simulink model "xTyTbeta1beta2"  (Simulink 10.0)
settings: Solver=FixedStepDiscrete  StartTime=0.0  StopTime=TF  FixedStep=5e-2  RelTol=1e-4  EnableMultiTasking=on
values from neighbouring files (symbols this model uses):
  Lb1 = 0.3    [s_robot_planare.m]
  Lb2 = 0.4    [s_robot_planare.m]
settings Model: Creator=prof. G. Celentano  LastModifiedBy=giuseppericcio
settings DataIOCC: LimitDataPoints=on  SignalLoggingSaveFormat=ModelDataLogs
settings OptimizationCC: ExpressionDepthLimit=2147483647  InitFltsAndDblsToZero=on
settings DebuggingCC: SaveWithParameterizedLinksMsg=none  SolverPrmCheckMsg=warning  FcnCallInpInsideContextMsg=warning  StateNameClashWarn=warning
settings GRTTargetCC: TargetFcnLib=ansi_tfl_tmw.mat

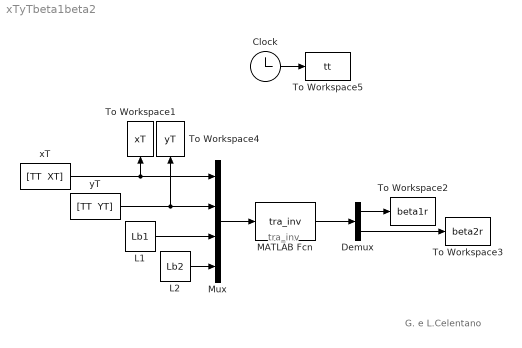
== system xTyTbeta1beta2 ==
  note: tra_inv
  note: G. e L.Celentano
  Clock : Clock
  Demux : Demux  Outputs=2
  L1 : Constant  Value=Lb1
  L2 : Constant  Value=Lb2
  MATLAB Fcn : MATLABFcn  MATLABFcn=tra_inv
  Mux : Mux
  To Workspace1 : ToWorkspace  VariableName=xT  SampleTime=-1
  To Workspace2 : ToWorkspace  VariableName=beta1r  SampleTime=-1
  To Workspace3 : ToWorkspace  VariableName=beta2r  SampleTime=-1
  To Workspace4 : ToWorkspace  VariableName=yT  SampleTime=-1
  To Workspace5 : ToWorkspace  VariableName=tt  SampleTime=-1
  xT : FromWorkspace  VariableName="[TT  XT]"  SampleTime=0
  yT : FromWorkspace  VariableName="[TT  YT]"  SampleTime=0
  wires:
  Mux/1 -> MATLAB Fcn/1
  xT/1 -> Mux/1, To Workspace1/1
  yT/1 -> Mux/2, To Workspace4/1
  MATLAB Fcn/1 -> Demux/1
  Demux/1 -> To Workspace2/1
  Demux/2 -> To Workspace3/1
  L1/1 -> Mux/3
  L2/1 -> Mux/4
  Clock/1 -> To Workspace5/1
